simulink model "edrive"  (R2016b)
settings: Solver=ode1  StartTime=0.0  StopTime=1  FixedStep=ctrlConst.TsSim  MaxStep=1e-6  RelTol=1e-3  EnableMultiTasking=on
PreLoadFcn:
  | %rtwdemo_pmsmfoc_data
StartFcn:
  | %clear executionProfile
StopFcn:
  | %try
  | %  AddExecutionProfileToDataInspector();
  | %end
undefined symbols (not defined in the file or in its folder): canChannel, ctrlConst, ECM, EGM, hm11, hm13, hm5, hm7, Np, pmsm, sensors, sldrtexcb_modeswitch, SpdSetTest, theta0, TrqSetTest, Ts_10ms, Tsw
libraries: powerlib x26, canmsglib x23, simulink x14, canlib x12, powerlib_extras x9
(part 1 of 4)
Description:
  | Field-Oriented Control of Permanent Magnet Synchronous Machine
  | 
  | Demonstrates a Field-Oriented Control algorithm with Space Vector Modulation for a Permanent Magnet Synchronous Machine (PMSM).
  | The test bench can be used to evaluate the system performance. Examples include turning the motor on, searching for a valid rotor position,
  | transitioning to closed loop operation, and changing speed and torque during closed loop control.
  | The Embedded Processor subsystem contains the controller algorithm (which supports C code generation) as well as simulation models of peripherals.
settings Model: Creator=The MathWorks, Inc.  LastModifiedBy=xingchun.zhang
settings SolverCC: ZeroCrossControl=DisableAll  InsertRTBMode=Never (minimum delay)
settings DataIOCC: LimitDataPoints=on  SaveFormat=Array  SignalLogging=off  DSMLogging=off  ReturnWorkspaceOutputsName=effEDrive
settings OptimizationCC: DefaultParameterBehavior=Inlined  UseDivisionForNetSlopeComputation=on  UseFloatMulNetSlope=on  DefaultUnderspecifiedDataType=single  InlineInvariantSignals=on  PassReuseOutputArgsAs=Individual arguments  ExpressionDepthLimit=2147483647  ZeroExternalMemoryAtStartup=off  ZeroInternalMemoryAtStartup=off  NoFixptDivByZeroProtection=on  EfficientFloat2IntCast=on  LifeSpan=1
settings DebuggingCC: ReadBeforeWriteMsg=DisableAll  WriteAfterWriteMsg=DisableAll  WriteAfterReadMsg=DisableAll  AlgebraicLoopMsg=none  MultiTaskDSMMsg=warning  SingleTaskRateTransMsg=error  IntegerOverflowMsg=none  ParameterPrecisionLossMsg=none  FcnCallInpInsideContextMsg=warning  UnconnectedInputMsg=none  UnconnectedOutputMsg=none  UnconnectedLineMsg=none  BusObjectLabelMismatch=none  AssertControl=DisableAll  AllowSymbolicDim=off  StateNameClashWarn=warning  SFUnexpectedBacktrackingDiag=warning  SFNoUnconditionalDefaultTransitionDiag=warning  SFExecutionAtInitializationDiag=none  IntegerSaturationMsg=none  UnitsInconsistencyMsg=none
settings HardwareCC: ProdBitPerPointer=32  ProdBitPerSizeT=32  ProdBitPerPtrDiffT=32  ProdLargestAtomicFloat=None  ProdWordSize=32  ProdHWDeviceType=Infineon->TriCore
settings ModelReferenceCC: UpdateModelReferenceTargets=IfOutOfDate  ModelReferenceNumInstancesAllowed=Single  PropagateSignalLabelsOutOfModel=off
settings SFSimCC: SFSimEcho=off
settings RTWCC: SystemTargetFile=ert.tlc  GenerateMakefile=off  TemplateMakefile=ec_target.tmf  Description=Embedded Coder  GenerateReport=on  RTWVerbose=off  CustomInclude=C:\MatlabWS\motorcontrol\sfun  IncludeHyperlinkInReport=on  LaunchReport=on  PortableWordSizes=on  CodeExecutionProfiling=on  CodeProfilingSaveOptions=AllData  CodeProfilingInstrumentation=on  GenerateTraceInfo=on  GenerateTraceReport=on  GenerateTraceReportSl=on  GenerateTraceReportSf=on  GenerateTraceReportEml=on  GenerateWebview=on  GenerateCodeMetricsReport=on
settings RTWCC: CustomSource=|
  | C:\MatlabWS\motorcontrol\sfun\C2SfunShell.h
  | C:\MatlabWS\motorcontrol\sfun\C2SfunShell.c
settings CodeAppCC: ForceParamTrailComments=on  IgnoreCustomStorageClasses=off  IgnoreTestpoints=on  MaxIdLength=64  SimulinkDataObjDesc=on  MATLABFcnDesc=on  CustomSymbolStrGlobalVar=rt$N$M  CustomSymbolStrType=$N$M  CustomSymbolStrFcn=$N$M$F  CustomSymbolStrFcnArg=$I$N$M  CustomSymbolStrMacro=$N$M  InsertBlockDesc=on  MATLABSourceComments=on  InternalIdentifier=Classic
settings ERTTargetCC: GeneratePreprocessorConditionals=Disable all  CombineSignalStateStructs=on  SupportAbsoluteTime=off  SupportNonFinite=off  SupportComplex=off  SupportNonInlinedSFcns=on  RemoveResetFunc=off  ParenthesesLevel=Maximum  InlinedParameterPlacement=NonHierarchical  ERTCustomFileTemplate=example_file_process.tlc  ERTFilePackagingFormat=CompactWithDataFile  ConvertIfToSwitch=off  SuppressUnreachableDefaultCases=off
settings ConfigComp: CovMetricSettings=dcmtrzow  CovHTMLOptions=-aTS=1 -bRG=1 -bTC=1 -hTR=0 -nFC=0 -scm=1 -bcm=1 -xEv=0  CovHtmlReporting=on  CovSaveCumulativeToWorkspaceVar=on  CovSaveSingleToWorkspaceVar=on  CovExternalEMLEnable=off  CovSFcnEnable=off

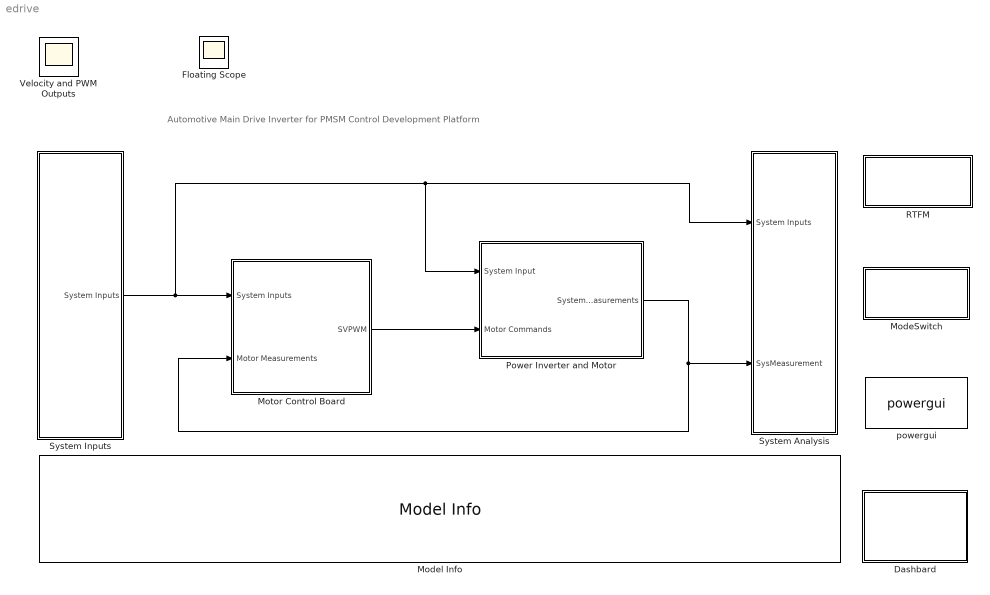
== system edrive ==
  note: Automotive Main Drive Inverter for PMSM Control
      | Development Platform
  Dashbard : Subsystem
  ModeSwitch : Subsystem  InitFcn=sldrtexcb_modeswitch('CheckKernel');  mask(Simulink Desktop Real-Time Example Mode Switch){}
      settings: OpenFcn=sldrtexcb_modeswitch(gcbh);
      mask Display: disp('Switch To\nExternal Mode');
  Model Info : simulink/Model-Wide Utilities/Model Info  Frame=on  DisplayStringWithTags=Model Description: %<Description>  HorizontalTextAlignment=Left  LeftAlignmentValue=0.02  SourceBlockDiagram=edrive  TagMaxNumber=20
  Motor Control Board : Subsystem
      mask Display: image('rtwdemo_pmsmfoc_processor.png')
  Power Inverter and Motor : Subsystem  Description=""
      mask Display: image('rtwdemo_pmsmfoc_motor.png')
  "RTFM " : Subsystem  mask(Simulink Desktop Real-Time Example Info){}
      settings: OpenFcn=web([docroot '/sldrt/examples/real-time-van-der-pol-simulation.html']);
      mask Display: disp('Info')
  System Analysis : Subsystem  Description=|
      | System Analysis for Speed Control Design
      | 
      | Analyize and plot signals used to analyize performance of
      | speed  control designs
      mask Display: fprintf('System\nAnalysis')
  System Inputs : Subsystem  Description=""  SystemSampleTime=10e-3
      mask Display: fprintf('System\nInputs')
  powergui : powerlib/powergui  Priority=1  SimulationMode=Discrete  SolverType=Tustin  SampleTime=ctrlConst.TsSimP  frequency=60  SPID=off  DisableSnubberDevices=off  DisableRonSwitches=off  DisableVfSwitches=off  SwTol=0  DisplayEquations=off  Interpol=off  ExternalGateDelay=off  methode=off  Ts=0  FunctionMessages=off  echomessages=off  HookPort=off  EnableUseOfTLC=off  x0status=blocks  frequencyindice=0  Pbase=100e6  ErrMax=1e-4  Iterations=50  UnitsV=kV  UnitsW=MW  buscounter=0  RestoreLinks=warning  ResistiveCurrentMeasurement=off  Frange=[0:2:500]  Ylog=off  Xlog=on  ShowGrid=off  save=off  variable=ZData  structure=ElecData  ZoomFFT=off  StartTime=0.482  cycles=10  DisplayStyle=2  fundamental=600  FreqAxis=off  MaxFrequency=10000  frequencyindicesteady=1  RmsSteady=1  display=off
  Floating Scope : Scope
  Velocity and PWM Outputs : Scope
  wires:
  Motor Control Board/1(SVPWM) -> Power Inverter and Motor/2(Motor Commands)
  System Inputs/1(System Inputs) -> Motor Control Board/1(System Inputs), System Analysis/1(System Inputs), Power Inverter and Motor/1(System Input)
  Power Inverter and Motor/1(System Measurements) -> Motor Control Board/2(Motor Measurements), System Analysis/2(SysMeasurement)

== system edrive/Dashbard ==
  Dashboard Scope : Subsystem  DialogController=hmiCreateDDGDialog  IsWebBlock=on  mask(MWDashboardBlock){webBlockId=dbaa0f85-305e-462e-a7a1-755dd39fbe0d, webBlockType=sdiscope, ShowInitialText=on, HMISrcModelName=edrive}
      mask prompts: webBlockId "WebBlock Id"; webBlockType "WebBlock Type"; HMISrcModelName "Source Model"
      mask help: SimulinkHMI:dialogs:HMIScopeDialogDesc
      mask Help: helpview([docroot '/mapfiles/simulink.map'], 'hmi_scope')
      mask Display:
      | if strcmp(get_param(bdroot(gcb),'BlockDiagramType'), 'library')
      |     image([(matlabroot) '/toolbox/simulink/hmi/icons/DashboardScope.png']);
      | end
  Gauge : Subsystem  DialogController=hmiCreateDDGDialog  IsWebBlock=on  mask(MWDashboardBlock){webBlockId=feaa2327-ad78-499e-96da-9991cfa67485, webBlockType=circulargauge, ShowInLibBrowser=on, ShowInitialText=on, HMISrcModelName=edrive}
      mask prompts: webBlockId "WebBlock Id"; webBlockType "WebBlock Type"; HMISrcModelName "Source Model"
      mask help: SimulinkHMI:dialogs:CircularGaugeDialogDesc
      mask Help: helpview([docroot '/mapfiles/simulink.map'], 'hmi_gauge')
      mask Display:
      | if strcmp(get_param(bdroot(gcb),'BlockDiagramType'), 'library')
      |     image([(matlabroot) '/toolbox/simulink/hmi/icons/CircularGauge.png']);
      | end
  Rotary Switch : Subsystem  DialogController=hmiCreateDDGDialog  IsWebBlock=on  mask(MWDashboardBlock){webBlockId=5f39aa38-4a9c-4792-be93-f8b3064abbd5, webBlockType=discreteknob, ShowInLibBrowser=on, ShowInitialText=on, HMISrcModelName=edrive}
      mask prompts: webBlockId "WebBlock Id"; webBlockType "WebBlock Type"; HMISrcModelName "Source Model"
      mask help: SimulinkHMI:dialogs:DiscreteKnobDialogDesc
      mask Help: helpview([docroot '/mapfiles/simulink.map'], 'hmi_rotary_switch')
      mask Display:
      | model = bdroot(gcb);
      | if strcmp(get_param(model,'BlockDiagramType'), 'library')
      |     image([(matlabroot) '/toolbox/simulink/hmi/icons/DiscreteKnob.png']);
      | end
  Slider : Subsystem  DialogController=hmiCreateDDGDialog  IsWebBlock=on  mask(MWDashboardBlock){webBlockId=79de6ff3-7337-4cfe-9aff-1e6db678eec5, webBlockType=slider, ShowInLibBrowser=on, ShowInitialText=on, HMISrcModelName=edrive}
      mask prompts: webBlockId "WebBlock Id"; webBlockType "WebBlock Type"; HMISrcModelName "Source Model"
      mask help: SimulinkHMI:dialogs:SliderDialogDesc
      mask Help: helpview([docroot '/mapfiles/simulink.map'], 'hmi_slider')
      mask Display:
      | if strcmp(get_param(bdroot(gcb),'BlockDiagramType'), 'library')
      |     image([(matlabroot) '/toolbox/simulink/hmi/icons/Slider.png']);
      | end

== system edrive/ModeSwitch ==

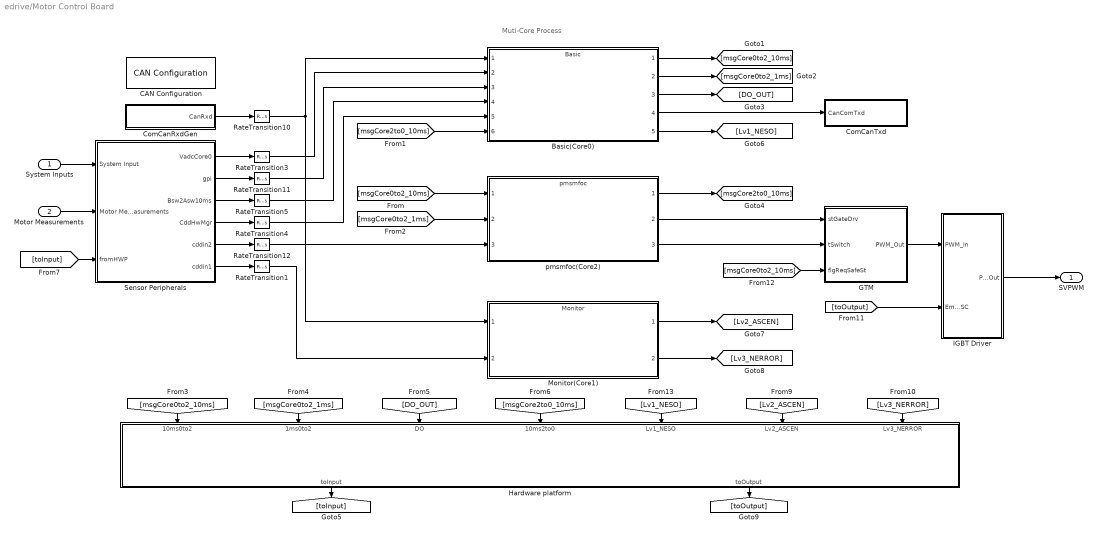
== system edrive/Motor Control Board ==
  note: Muti-Core Process
  System Inputs : Inport
  Motor Measurements : Inport  Port=2
  Basic(Core0) : ModelReference  ModelNameDialog=Basic.slx  SimulationMode=Normal  ModelReferenceVersion=1.11689
  CAN Configuration : canlib/CAN Configuration  BlockHandle=7528.001  DeviceMenu=(none)  Device=Kvaser Virtual 1 (Channel 1)  ObjConstructor=canChannel('Kvaser', 'Virtual 1', 1)  BusSpeed=500000  EnableBitParameters=off  SJW=1  TSEG1=4  TSEG2=3  NSamples=1  AckMode=Normal
  ComCanRxdGen : Subsystem
  ComCanTxd : Subsystem
  GTM : Subsystem  SystemSampleTime=Tsw
  Hardware platform : Subsystem  SystemSampleTime=Tsw
  IGBT Driver : Subsystem  SystemSampleTime=Tsw
  Monitor(Core1) : ModelReference  ModelNameDialog=Monitor.slx  SimulationMode=Normal  ModelReferenceVersion=1.8110
  RateTransition{1,3..5,10..12} (7 alike) : RateTransition
  Sensor Peripherals : Subsystem  Description=|
      | Elaborate Sensor Models
      | 
      | ADC and QEP and Encoder Models
  pmsmfoc(Core2) : ModelReference  ModelNameDialog=pmsmfoc.slx  SimulationMode=Normal  ModelReferenceVersion=1.9399
      settings: AttributesFormatString=|
      | -----------------------------
      | Sample rate: ctrlConst.TsSwitch
  SVPWM : Outport
  wires:
  System Inputs/1 -> Sensor Peripherals/1(System Input)
  Motor Measurements/1 -> Sensor Peripherals/2(Motor Measurements)
  ComCanRxdGen/1(CanRxd) -> RateTransition10/1
  Sensor Peripherals/2(gpi) -> RateTransition11/1
  Sensor Peripherals/5(cddin2) -> RateTransition12/1
  RateTransition12/1 -> pmsmfoc(Core2)/3
  RateTransition10/1 -> Monitor(Core1)/1, Basic(Core0)/1
  RateTransition11/1 -> Basic(Core0)/3
  pmsmfoc(Core2)/1 -> [msgCore2to0_10ms]
  pmsmfoc(Core2)/3 -> GTM/2(tSwitch)
  Basic(Core0)/1 -> [msgCore0to2_10ms]
  Sensor Peripherals/1(VadcCore0) -> RateTransition3/1
  Sensor Peripherals/6(cddin1) -> RateTransition1/1
  RateTransition1/1 -> Monitor(Core1)/2
  RateTransition3/1 -> Basic(Core0)/2
  [msgCore0to2_10ms] -> pmsmfoc(Core2)/1
  Basic(Core0)/2 -> [msgCore0to2_1ms]
  [msgCore0to2_1ms] -> pmsmfoc(Core2)/2
  [msgCore2to0_10ms] -> Basic(Core0)/6
  IGBT Driver/1(PWM_Out) -> SVPWM/1
  GTM/1(PWM_Out) -> IGBT Driver/1(PWM_In)
  Sensor Peripherals/4(CddHwMgr) -> RateTransition4/1
  RateTransition4/1 -> Basic(Core0)/5
  Sensor Peripherals/3(Bsw2Asw10ms) -> RateTransition5/1
  RateTransition5/1 -> Basic(Core0)/4
  pmsmfoc(Core2)/2 -> GTM/1(stGateDrv)
  Basic(Core0)/3 -> [DO_OUT]
  [msgCore0to2_10ms] -> Hardware platform/1(10ms0to2)
  [msgCore0to2_1ms] -> Hardware platform/2(1ms0to2)
  [DO_OUT] -> Hardware platform/3(DO)
  [msgCore2to0_10ms] -> Hardware platform/4(10ms2to0)
  Hardware platform/1(toInput) -> [toInput]
  [toInput] -> Sensor Peripherals/3(fromHWP)
  [Lv2_ASCEN] -> Hardware platform/6(Lv2_ASCEN)
  [Lv3_NERROR] -> Hardware platform/7(Lv3_NERROR)
  Hardware platform/2(toOutput) -> [toOutput]
  [toOutput] -> IGBT Driver/2(Emgy_ASC)
  [msgCore0to2_10ms] -> GTM/3(flgReqSafeSt)
  Basic(Core0)/4 -> ComCanTxd/1(CanComTxd)
  [Lv1_NESO] -> Hardware platform/5(Lv1_NESO)
  Basic(Core0)/5 -> [Lv1_NESO]
  Monitor(Core1)/1 -> [Lv2_ASCEN]
  Monitor(Core1)/2 -> [Lv3_NERROR]

== system edrive/Power Inverter and Motor ==
  note: Models the PMSM motor and inverter power electronics
      | Outputs electrical and mechanical measurements.
  note: Inverter and Motor
  System Input : Inport
  Motor Commands : Inport  Port=2
  Bus Creator : BusCreator  Inputs=3
  Bus Selector : BusSelector  OutputSignals=MotorMode,Load
  Inverter : Subsystem
  Motor_feishi150 : Subsystem
  System Measurements : Outport
  wires:
  Inverter/1("EleMeasurement ") -> Bus Creator/1  "electrical_measurements"
  Bus Creator/1 -> System Measurements/1
  Motor_feishi150/1(MotorMeasure) -> Bus Creator/2  "mechanical_measurements"
  System Input/1 -> Bus Selector/1
  Bus Selector/2 -> Motor_feishi150/2(Speed or Torque)  "<Load>"
  Motor Commands/1 -> Bus Creator/3, Inverter/1(gate1)
  Bus Selector/1 -> Motor_feishi150/1(MotorMode)  "<MotorMode>"
  connections:
  Motor_feishi150/LConn2 -- Inverter/RConn2
  Motor_feishi150/LConn1 -- Inverter/RConn1
  Motor_feishi150/LConn3 -- Inverter/RConn3

== system edrive/RTFM  ==

== system edrive/System Analysis ==
  note: System Analysis
  note: Visualize common signals of interest.
  System Inputs : Inport
  SysMeasurement : Inport  Port=2
  Bus Creator1 : BusCreator  Inputs=2
  Bus Selector4 : BusSelector  OutputSignals=Torque
  Data Type Conversion : DataTypeConversion  OutDataTypeStr=double
  Measure : Subsystem
  PMSM Drive : Scope  NumInputPorts=6
  Pass or not : Display
  System test : Subsystem
  effEDrive : Scope
  wires:
  SysMeasurement/1 -> Measure/1(motor)
  Bus Creator1/1 -> PMSM Drive/1, System test/1(torque_in)  "Torque"
  Measure/2(speed) -> PMSM Drive/2  "Speed"
  Measure/3(Current) -> PMSM Drive/3  "Is,iq,id"
  Measure/4(Voltage) -> PMSM Drive/4  "vs,vq,vd"
  Measure/5(Power) -> PMSM Drive/5  "Power"
  System test/1(Out) -> Pass or not/1
  System Inputs/1 -> Bus Selector4/1
  Bus Selector4/1 -> Data Type Conversion/1  "<Torque>"
  Measure/1(Torque) -> Bus Creator1/2  "TorqueAct"
  [ModeInCan] -> PMSM Drive/6
  Measure/6(effEDrive) -> effEDrive/1
  Data Type Conversion/1 -> Bus Creator1/1

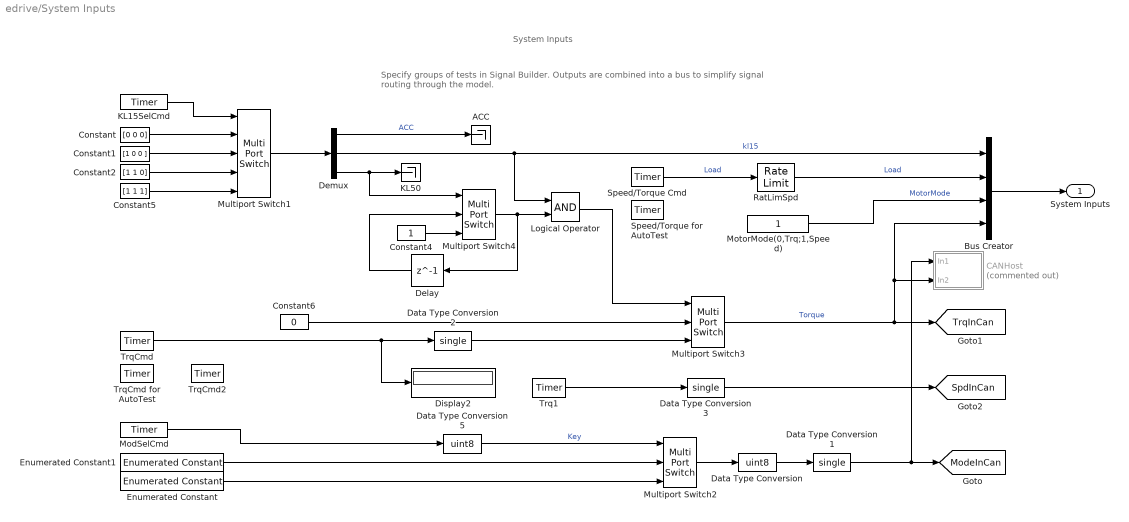
== system edrive/System Inputs ==
  note: System Inputs
  note: Specify groups of tests in Signal Builder. Outputs are combined into a bus
      | to simplify signal routing through the model.
  ACC : Terminator
  Bus Creator : BusCreator  Inputs=4
  CANHost : Subsystem  Commented=on
  Constant : Constant  Value=[0 0 0]  OutDataTypeStr=boolean
  Constant1 : Constant  Value=[1 0 0 ]  OutDataTypeStr=boolean
  Constant2 : Constant  Value=[1 1 0]  OutDataTypeStr=boolean
  Constant4 : Constant  OutDataTypeStr=boolean
  Constant5 : Constant  Value=[1 1 1]  OutDataTypeStr=boolean
  Constant6 : Constant  Value=0  OutDataTypeStr=single
  Data Type Conversion : DataTypeConversion  OutDataTypeStr=uint8
  Data Type Conversion1 : DataTypeConversion  OutDataTypeStr=single
  Data Type Conversion2 : DataTypeConversion  OutDataTypeStr=single
  Data Type Conversion3 : DataTypeConversion  OutDataTypeStr=single
  Data Type Conversion5 : DataTypeConversion  OutDataTypeStr=uint8  ConvertRealWorld=Stored Integer (SI)
  Delay : Delay  DelayLength=1  InitialCondition=0
  Demux : Demux  Outputs=3
  Display2 : Display
  Enumerated Constant : simulink/Sources/Enumerated Constant  OutDataTypeStr=Enum: ECM  Value=ECM.TrqCtrl  SampleTime=inf
  Enumerated Constant1 : simulink/Sources/Enumerated Constant  OutDataTypeStr=Enum: ECM  Value=ECM.Standby  SampleTime=inf
  KL15SelCmd : powerlib_extras/Control  Blocks/Timer  t="[ 0  0.03  0.1  0.2 0.9]"  e="[3  3  3  3 3]"
  KL50 : Terminator
  Logical Operator : Logic  AllPortsSameDT=off  OutDataTypeStr=boolean
  ModSelCmd : powerlib_extras/Control  Blocks/Timer  t="[ 0  0.1  0.2  0.3 0.4]"  e="[0  0  1  1 1]"
  MotorMode(0,Trq;1,Speed) : Constant  OutDataTypeStr=double
  Multiport Switch1 : MultiPortSwitch  DataPortOrder=Zero-based contiguous  Inputs=4
  Multiport Switch2 : MultiPortSwitch  DataPortOrder=Zero-based contiguous  Inputs=2
  Multiport Switch3 : MultiPortSwitch  DataPortOrder=Zero-based contiguous  Inputs=2
  Multiport Switch4 : MultiPortSwitch  DataPortOrder=Zero-based contiguous  Inputs=2
  RatLimSpd : RateLimiter  RisingSlewLimit=5000  FallingSlewLimit=-5000  LinearizeAsGain=off
  Speed/Torque Cmd : powerlib_extras/Control  Blocks/Timer  t="[ 0  0.05  0.25  0.4]"  e="[3  3  3  15]*(1000)"
  Speed/Torque for AutoTest : powerlib_extras/Control  Blocks/Timer  t="[ 0  0.1  0.25  0.5]"  e="[1  1  1  1]*SpdSetTest"
  Trq1 : powerlib_extras/Control  Blocks/Timer  t="[ 0  0.1  0.2  0.5]"  e="[0  0  2000  2000]*2"
  TrqCmd : powerlib_extras/Control  Blocks/Timer  t="[ 0  0.2 0.25 0.3 0.7 0.8]"  e="[ 0  0  0   1   1  1]*(200)"
  TrqCmd for AutoTest : powerlib_extras/Control  Blocks/Timer  t="[ 0  0.06  0.099 0.15]"  e="[ 0  1 1 1]*TrqSetTest"
  TrqCmd2 : powerlib_extras/Control  Blocks/Timer  t="[ 0  1  1.1  1.2 1.3 1.4 1.5 1.6 1.7 1.8 1.9 2.0 2.1 2.2 2.3 2.4 2.5 2.6 2.7 2.8 2.9]"  e=[ 0 1 2 3 4 5 6 7 8 9 10 11 12 13 14 15 16 17 18 19 20]*20
  System Inputs : Outport
  tag scope: ModeInCan=global, SpdInCan=global, TrqInCan=global
  wires:
  Constant/1 -> Multiport Switch1/2
  Multiport Switch1/1 -> Demux/1
  Enumerated Constant1/1 -> Multiport Switch2/2
  Multiport Switch2/1 -> Data Type Conversion/1
  Multiport Switch3/1 -> Bus Creator/4, CANHost/2(In2), [TrqInCan]  "Torque"
  Multiport Switch4/1 -> Logical Operator/2, Delay/1
  Delay/1 -> Multiport Switch4/2
  Constant4/1 -> Multiport Switch4/3
  Logical Operator/1 -> Multiport Switch3/1
  Constant1/1 -> Multiport Switch1/3
  Constant2/1 -> Multiport Switch1/4
  Demux/3 -> Multiport Switch4/1, KL50/1
  Demux/1 -> ACC/1  "ACC"
  Constant6/1 -> Multiport Switch3/2
  Demux/2 -> Bus Creator/1, Logical Operator/1  "kl15"
  Bus Creator/1 -> System Inputs/1
  Speed/Torque Cmd/1 -> RatLimSpd/1  "Load"
  Data Type Conversion/1 -> Data Type Conversion1/1
  Data Type Conversion1/1 -> CANHost/1(In1), [ModeInCan]
  Constant5/1 -> Multiport Switch1/5
  Data Type Conversion2/1 -> Multiport Switch3/3
  Trq1/1 -> Data Type Conversion3/1
  Data Type Conversion3/1 -> [SpdInCan]
  MotorMode(0,Trq;1,Speed)/1 -> Bus Creator/3  "MotorMode"
  RatLimSpd/1 -> Bus Creator/2  "Load"
  ModSelCmd/1 -> Data Type Conversion5/1
  Enumerated Constant/1 -> Multiport Switch2/3
  KL15SelCmd/1 -> Multiport Switch1/1
  Data Type Conversion5/1 -> Multiport Switch2/1  "Key"
  TrqCmd/1 -> Display2/1, Data Type Conversion2/1

== system edrive/Dashbard/Dashboard Scope ==

== system edrive/Dashbard/Gauge ==

== system edrive/Dashbard/Rotary Switch ==

== system edrive/Dashbard/Slider ==

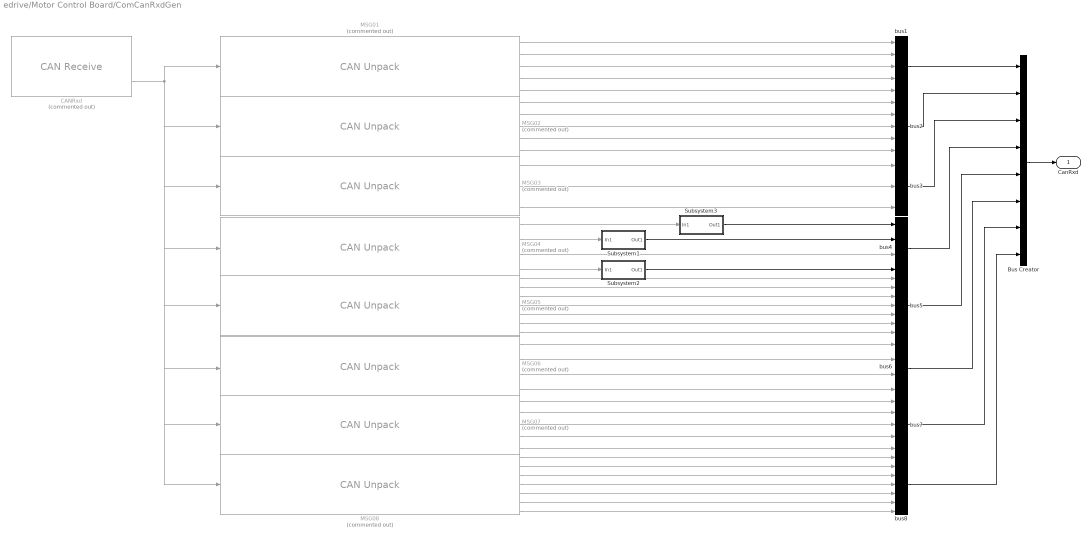
== system edrive/Motor Control Board/ComCanRxdGen ==
  Bus Creator : BusCreator  Inputs=8  OutDataTypeStr=Bus: CANRXDST
  CANRxd : canlib/CAN Receive  Commented=on  BlockHandle=7531.0005  DeviceMenu=Kvaser Virtual 1 (Channel 1)  Device=Kvaser Virtual 1 (Channel 1)  ObjConstructor=canChannel('Kvaser', 'Virtual 1', 1)  EnableStandardIDsFilter=off  StandardIDs=0  EnableExtendedIDsFilter=off  ExtendedIDs=0  SampleTime=0.01  MsgsPerTimestep=all  StdIDsCombo=Allow all  ExtIDsCombo=Allow all  InternalFilterUpdateStatus=off
  MSG01 : canmsglib/CAN Unpack  Commented=on  CANdbFile=C:\MatlabWS\motorcontrol\controller\CAN_COM.dbc  MsgList=MSG_01  MsgName=MSG_01  MsgIDType=Standard (11-bit identifier)  MsgIdentifier=768  MsgLength=8  SignalInfo=MSG01_IdcMax$0$0$0$4$4$4$4$4$4$4$#MSG01_IdcMin$0$0$0$4$4$4$4$4$4$4$#MSG01_UdcMax$0$0$0$4$4$4$4$4$4$4$#MSG01_UdcMin$0$0$0$4$4$4$4$4$4$4$#MSG01_stHvbMaiRly$0$0$0$4$4$4$4$4$4$4$#  NSignals=5  IDPort=off  TimestampPort=off  ErrorPort=off  RemotePort=off  LengthPort=off  StatusPort=off  StartBits=0  SignalSizes=0  ByteOrders=0  DataTypes=0  MultiplexTypes=0  MultiplexValues=0  Factors=0  Offsets=0  Minimums=0  Maximums=0
      settings: DataFormat=CANdb specified signals
  MSG02 : canmsglib/CAN Unpack  Commented=on  CANdbFile=C:\MatlabWS\motorcontrol\controller\CAN_COM.dbc  MsgList=MSG_02  MsgName=MSG_02  MsgIDType=Standard (11-bit identifier)  MsgIdentifier=784  MsgLength=8  SignalInfo=MSG02_KpHigh$0$0$0$4$4$4$4$4$4$4$#MSG02_KpLow$0$0$0$4$4$4$4$4$4$4$#MSG02_NDeltaBound$0$0$0$4$4$4$4$4$4$4$#MSG02_TrqPAmax$0$0$0$4$4$4$4$4$4$4$#MSG02_TrqPAmin$0$0$0$4$4$4$4$4$4$4$#  NSignals=5  IDPort=off  TimestampPort=off  ErrorPort=off  RemotePort=off  LengthPort=off  StatusPort=off  StartBits=0  SignalSizes=0  ByteOrders=0  DataTypes=0  MultiplexTypes=0  MultiplexValues=0  Factors=0  Offsets=0  Minimums=0  Maximums=0
      settings: DataFormat=CANdb specified signals
  MSG03 : canmsglib/CAN Unpack  Commented=on  CANdbFile=C:\MatlabWS\motorcontrol\controller\CAN_COM.dbc  MsgList=MSG_03  MsgName=MSG_03  MsgIDType=Standard (11-bit identifier)  MsgIdentifier=800  MsgLength=8  SignalInfo=MSG03_TrqMax$0$0$0$4$4$4$4$4$4$4$#MSG03_TrqMin$0$0$0$4$4$4$4$4$4$4$#MSG03_cTrqSlopeMax$0$0$0$4$4$4$4$4$4$4$#  NSignals=3  IDPort=off  TimestampPort=off  ErrorPort=off  RemotePort=off  LengthPort=off  StatusPort=off  StartBits=0  SignalSizes=0  ByteOrders=0  DataTypes=0  MultiplexTypes=0  MultiplexValues=0  Factors=0  Offsets=0  Minimums=0  Maximums=0
      settings: DataFormat=CANdb specified signals
  MSG04 : canmsglib/CAN Unpack  Commented=on  CANdbFile=C:\MatlabWS\motorcontrol\controller\CAN_COM.dbc  MsgList=MSG_04  MsgName=MSG_04  MsgIDType=Standard (11-bit identifier)  MsgIdentifier=256  MsgLength=8  SignalInfo=MSG04_NSetP$0$0$0$4$4$4$4$4$4$4$#MSG04_TrqSetP$0$0$0$4$4$4$4$4$4$4$#MSG04_UdcSetP$0$0$0$4$4$4$4$4$4$4$#MSG04_stModeReq$0$0$0$4$4$4$4$4$4$4$#  NSignals=4  IDPort=off  TimestampPort=off  ErrorPort=off  RemotePort=off  LengthPort=off  StatusPort=off  StartBits=0  SignalSizes=0  ByteOrders=0  DataTypes=0  MultiplexTypes=0  MultiplexValues=0  Factors=0  Offsets=0  Minimums=0  Maximums=0
      settings: DataFormat=CANdb specified signals
  MSG05 : canmsglib/CAN Unpack  Commented=on  CANdbFile=C:\MatlabWS\motorcontrol\controller\CAN_COM.dbc  MsgList=MSG_05  MsgName=MSG_05  MsgIDType=Standard (11-bit identifier)  MsgIdentifier=272  MsgLength=8  SignalInfo=MSG05_FrqStrSetP$0$0$0$4$4$4$4$4$4$4$#MSG05_IsSetP$0$0$0$4$4$4$4$4$4$4$#MSG05_OfsAl$0$0$0$4$4$4$4$4$4$4$#MSG05_PumpCtl$0$0$0$4$4$4$4$4$4$4$#MSG05_bSetOfsAl$0$0$0$4$4$4$4$4$4$4$#MSG05_bUseFrqStrSynt$0$0$0$4$4$4$4$4$4$4$#MSG05_flgInvrCanActvnCmd$0$0$0$4$4$4$4$4$4$4$#  NSignals=7  IDPort=off  TimestampPort=off  ErrorPort=off  RemotePort=off  LengthPort=off  StatusPort=off  StartBits=0  SignalSizes=0  ByteOrders=0  DataTypes=0  MultiplexTypes=0  MultiplexValues=0  Factors=0  Offsets=0  Minimums=0  Maximums=0
      settings: DataFormat=CANdb specified signals
  MSG06 : canmsglib/CAN Unpack  Commented=on  CANdbFile=C:\MatlabWS\motorcontrol\controller\CAN_COM.dbc  MsgList=MSG_06  MsgName=MSG_06  MsgIDType=Standard (11-bit identifier)  MsgIdentifier=288  MsgLength=8  SignalInfo=MSG06_TrqDmpLim$0$0$0$4$4$4$4$4$4$4$#MSG06_TrqDmpMax$0$0$0$4$4$4$4$4$4$4$#MSG06_kDmp$0$0$0$4$4$4$4$4$4$4$#MSG06_stDstCReq$0$0$0$4$4$4$4$4$4$4$#  NSignals=4  IDPort=off  TimestampPort=off  ErrorPort=off  RemotePort=off  LengthPort=off  StatusPort=off  StartBits=0  SignalSizes=0  ByteOrders=0  DataTypes=0  MultiplexTypes=0  MultiplexValues=0  Factors=0  Offsets=0  Minimums=0  Maximums=0
      settings: DataFormat=CANdb specified signals
  MSG07 : canmsglib/CAN Unpack  Commented=on  CANdbFile=C:\MatlabWS\motorcontrol\controller\CAN_COM.dbc  MsgList=MSG_07  MsgName=CAN Msg  MsgIDType=Standard (11-bit identifier)  MsgIdentifier=0  MsgLength=8  SignalInfo=MSG07_IdcHvSetP$0$0$0$4$4$4$4$4$4$4$#MSG07_IdcLvSetP$0$0$0$4$4$4$4$4$4$4$#MSG07_UdcHvSetP$0$0$0$4$4$4$4$4$4$4$#MSG07_UdcLvSetP$0$0$0$4$4$4$4$4$4$4$#MSG07_stModeReq$0$0$0$4$4$4$4$4$4$4$#  NSignals=5  IDPort=off  TimestampPort=off  ErrorPort=off  RemotePort=off  LengthPort=off  StatusPort=off  StartBits=0  SignalSizes=0  ByteOrders=0  DataTypes=0  MultiplexTypes=0  MultiplexValues=0  Factors=0  Offsets=0  Minimums=0  Maximums=0
      settings: DataFormat=CANdb specified signals
  MSG08 : canmsglib/CAN Unpack  Commented=on  CANdbFile=C:\MatlabWS\motorcontrol\controller\CAN_COM.dbc  MsgList=MSG_08  MsgName=CAN Msg  MsgIDType=Standard (11-bit identifier)  MsgIdentifier=0  MsgLength=8  SignalInfo=MSG08_Alpha_Voltage_Cmd$0$0$0$4$4$4$4$4$4$4$#MSG08_Beta_Voltage_Cmd$0$0$0$4$4$4$4$4$4$4$#MSG08_D_Current_Cmd$0$0$0$4$4$4$4$4$4$4$#MSG08_D_Voltage_Cmd$0$0$0$4$4$4$4$4$4$4$#MSG08_Q_Current_Cmd$0$0$0$4$4$4$4$4$4$4$#MSG08_Q_Volatge_Cmd$0$0$0$4$4$4$4$4$4$4$#MSG08_control_mode$0$0$0$4$4$4$4$4$4$4$#  NSignals=7  IDPort=off  TimestampPort=off  ErrorPort=off  RemotePort=off  LengthPort=off  StatusPort=off  StartBits=0  SignalSizes=0  ByteOrders=0  DataTypes=0  MultiplexTypes=0  MultiplexValues=0  Factors=0  Offsets=0  Minimums=0  Maximums=0
      settings: DataFormat=CANdb specified signals
  Subsystem1 : Subsystem
  Subsystem2 : Subsystem
  Subsystem3 : Subsystem
  bus1 : BusCreator  Inputs=5  OutDataTypeStr=Bus: msg_MSG_01
  bus2 : BusCreator  Inputs=5  OutDataTypeStr=Bus: msg_MSG_02
  bus3 : BusCreator  Inputs=3  OutDataTypeStr=Bus: msg_MSG_03
  bus4 : BusCreator  Inputs=4  OutDataTypeStr=Bus: msg_MSG_04
  bus5 : BusCreator  Inputs=7  OutDataTypeStr=Bus: msg_MSG_05
  bus6 : BusCreator  Inputs=4  OutDataTypeStr=Bus: msg_MSG_06
  bus7 : BusCreator  Inputs=5  OutDataTypeStr=Bus: msg_MSG_07
  bus8 : BusCreator  Inputs=7  OutDataTypeStr=Bus: msg_MSG_08
  CanRxd : Outport  OutDataTypeStr=Bus: CANRXDST
  wires:
  Bus Creator/1 -> CanRxd/1
  MSG01/1 -> bus1/1
  MSG01/2 -> bus1/2
  MSG01/3 -> bus1/3
  MSG01/4 -> bus1/4
  MSG01/5 -> bus1/5
  CANRxd/2 -> MSG01/1, MSG02/1, MSG03/1, MSG04/1, MSG05/1, MSG06/1, MSG07/1, MSG08/1
  MSG02/1 -> bus2/1
  MSG02/2 -> bus2/2
  MSG02/3 -> bus2/3
  MSG02/4 -> bus2/4
  MSG02/5 -> bus2/5
  MSG03/1 -> bus3/1
  MSG03/2 -> bus3/2
  MSG04/1 -> Subsystem3/1(In1)
  MSG04/2 -> Subsystem1/1(In1)
  MSG04/3 -> bus4/3
  MSG04/4 -> Subsystem2/1(In1)
  MSG05/1 -> bus5/1
  MSG05/2 -> bus5/2
  MSG05/3 -> bus5/3
  MSG05/4 -> bus5/4
  MSG05/5 -> bus5/5
  MSG05/6 -> bus5/6
  MSG05/7 -> bus5/7
  MSG06/1 -> bus6/1
  MSG06/2 -> bus6/2
  MSG06/3 -> bus6/3
  MSG06/4 -> bus6/4
  MSG07/1 -> bus7/1
  MSG07/2 -> bus7/2
  MSG07/3 -> bus7/3
  MSG07/4 -> bus7/4
  MSG07/5 -> bus7/5
  MSG08/1 -> bus8/1
  MSG08/2 -> bus8/2
  MSG08/3 -> bus8/3
  MSG08/4 -> bus8/4
  MSG08/5 -> bus8/5
  MSG08/6 -> bus8/6
  MSG08/7 -> bus8/7
  MSG03/3 -> bus3/3
  Subsystem1/1(Out1) -> bus4/2
  Subsystem2/1(Out1) -> bus4/4
  bus1/1 -> Bus Creator/1
  bus2/1 -> Bus Creator/2
  bus3/1 -> Bus Creator/3
  bus4/1 -> Bus Creator/4
  bus5/1 -> Bus Creator/5
  bus6/1 -> Bus Creator/6
  bus7/1 -> Bus Creator/7
  bus8/1 -> Bus Creator/8
  Subsystem3/1(Out1) -> bus4/1

== system edrive/Motor Control Board/ComCanTxd ==
  CanComTxd : Inport  OutDataTypeStr=Bus: CANTXDST  SampleTime=Ts_10ms
  Bus Selector1 : BusSelector  OutputSignals=msg_EM_01,msg_EM_02,msg_EM_03,msg_EM_04,msg_EM_05,msg_EM_06,msg_EM_07
  Bus Selector2 : BusSelector  OutputSignals=EM01_IdcCurr,EM01_IsCurr,EM01_NCurr,EM01_TrqCurr,EM01_UdcCurr,EM01_stMode
  Bus Selector3 : BusSelector  OutputSignals=EM02_DBCTempU,EM02_DBCTempV,EM02_DBCTempW,EM02_TempCurrIGBT,EM02_TempCurrMot,EM02_TempCurrRotor,EM02_UT30Curr,EM02_bDernOvrIdc,EM02_bDernOvrUdc,EM02_bDernTemp,EM02_bDernTrqMax,EM02_bDernTrqMin,EM02_bDernUndrIdc,EM02_bDernUndrUdc,EM02_bDiagReq,EM02_bDstCActv,EM02_bReadyHv
  Bus Selector4 : BusSelector  OutputSignals=EM03_TempCurrCool,EM03_TempCurrDde,EM03_TrqAbsMax,EM03_TrqAbsMin,EM03_TrqCurrWoDstC,EM03_stGateDrv,EM03_stTrqEmMax,EM03_stTrqEmMin
  Bus Selector5 : BusSelector  OutputSignals=EM04_Isd,EM04_Isq,EM04_OfsAl,EM04_TempCurrPCB,EM04_agRtrElecSnsr
  Bus Selector6 : BusSelector  OutputSignals=EM05_FailCode1,EM05_FailCode2,EM05_FailCode3,EM05_FailCode4
  Bus Selector7 : BusSelector  OutputSignals=EM06_CodeVer,EM06_DataVer
  Bus Selector8 : BusSelector  OutputSignals=EM07_InterlockVtg,EM07_NCANSet,EM07_PumpVtg
  CAN Transmit : canlib/CAN Transmit  BlockHandle=7641.0006  DeviceMenu=(none)  Device=Kvaser Virtual 1 (Channel 1)  ObjConstructor=canChannel('Kvaser', 'Virtual 1', 1)  EnablePeriodicTransmit=off  MessagePeriod=1.000
  EM1 : canmsglib/CAN Pack  CANdbFile=C:\MatlabWS\motorcontrol\controller\CAN_COM.dbc  MsgList=EM_01  MsgName=EM_01  MsgIDType=Standard (11-bit identifier)  MsgIdentifier=512  MsgLength=8  SignalInfo=EM01_IdcCurr$32$11$1$2$1$0$1$-1023$-1023$1024$#EM01_IsCurr$53$11$1$2$1$0$5.000000e-01$0$0$1.023500e+03$#EM01_NCurr$16$16$1$2$1$0$1$-32767$-32767$32768$#EM01_TrqCurr$0$11$1$2$1$0$1$-1023$-1023$1024$#EM01_UdcCurr$43$10$1$2$1$0$1$0$0$1023$#EM01_stMode$11$4$1$2$1$0$1$0$0$15$#  NSignals=6  StartBits=str2num('[int32(32);int32(53);int32(16);int32(0);int32(43);int32(11)]')  SignalSizes=str2num('[int32(11);int32(11);int32(16);int32(11);int32(10);int32(4)]')  ByteOrders=str2num('[int32(1);int32(1);int32(1);int32(1);int32(1);int32(1)]')  DataTypes=str2num('[int32(2);int32(2);int32(2);int32(2);int32(2);int32(2)]')  MultiplexTypes=str2num('[int32(1);int32(1);int32(1);int32(1);int32(1);int32(1)]')  MultiplexValues=str2num('[double(0);double(0);double(0);double(0);double(0);double(0)]')  Factors=str2num('[double(1);double(5.000000e-01);double(1);double(1);double(1);double(1)]')  Offsets=str2num('[double(-1023);double(0);double(-32767);double(-1023);double(0);double(0)]')  Minimums=str2num('[double(-1023);double(0);double(-32767);double(-1023);double(0);double(0)]')  Maximums=str2num('[double(1024);double(1.023500e+03);double(32768);double(1024);double(1023);double(15)]')  Remote=off
      settings: DataFormat=CANdb specified signals
  EM2 : canmsglib/CAN Pack  CANdbFile=C:\MatlabWS\motorcontrol\controller\CAN_COM.dbc  MsgList=EM_02  MsgName=EM_02  MsgIDType=Standard (11-bit identifier)  MsgIdentifier=1024  MsgLength=8  SignalInfo=EM02_DBCTempU$24$8$1$2$1$0$1$-40$-40$215$#EM02_DBCTempV$32$8$1$2$1$0$1$-40$-40$215$#EM02_DBCTempW$40$8$1$2$1$0$1$-40$-40$215$#EM02_TempCurrIGBT$16$8$1$2$1$0$1$-40$-40$215$#EM02_TempCurrMot$0$8$1$2$1$0$1$-40$-40$215$#EM02_TempCurrRotor$8$8$1$2$1$0$1$-40$-40$215$#EM02_UT30Curr$58$6$1$2$1$0$5.000000e-01$0$0$3.150000e+01$#EM02_bDernOvrIdc$50$1$1$2$1$0$1$0$0$1$#EM02_bDernOvrUdc$48$1$1$2$1$0$1$0$0$1$#EM02_bDernTemp$52$1$1$2$1$0$1$0$0$1$#EM02_bDernTrqMax$55$1$1$2$1$0$1$0$0$1$#EM02_bDernTrqMin$54$1$1$2$1$0$1$0$0$1$#EM02_bDernUndrIdc$51$1$1$2$1$0$1$0$0$1$#EM02_bDernUndrUdc$49$1$1$2$1$0$1$0$0$1$#EM02_bDiagReq$53$1$1$2$1$0$1$0$0$1$#EM02_bDstCActv$56$1$1$2$1$0$1$0$0$1$#EM02_bReadyHv$57$1$1$2$1$0$1$0$0$1$#  NSignals=17  StartBits=str2num('[int32(24);int32(32);int32(40);int32(16);int32(0);int32(8);int32(58);int32(50);int32(48);int32(52);int32(55);int32(54);int32(51);int32(49);int32(53);int32(56);int32(57)]')  SignalSizes=str2num('[int32(8);int32(8);int32(8);int32(8);int32(8);int32(8);int32(6);int32(1);int32(1);int32(1);int32(1);int32(1);int32(1);int32(1);int32(1);int32(1);int32(1)]')  ByteOrders=str2num('[int32(1);int32(1);int32(1);int32(1);int32(1);int32(1);int32(1);int32(1);int32(1);int32(1);int32(1);int32(1);int32(1);int32(1);int32(1);int32(1);int32(1)]')  DataTypes=str2num('[int32(2);int32(2);int32(2);int32(2);int32(2);int32(2);int32(2);int32(2);int32(2);int32(2);int32(2);int32(2);int32(2);int32(2);int32(2);int32(2);int32(2)]')  MultiplexTypes=str2num('[int32(1);int32(1);int32(1);int32(1);int32(1);int32(1);int32(1);int32(1);int32(1);int32(1);int32(1);int32(1);int32(1);int32(1);int32(1);int32(1);int32(1)]')  MultiplexValues=str2num('[double(0);double(0);double(0);double(0);double(0);double(0);double(0);double(0);double(0);double(0);double(0);double(0);double(0);double(0);double(0);double(0);double(0)]')  Factors=str2num('[double(1);double(1);double(1);double(1);double(1);double(1);double(5.000000e-01);double(1);double(1);double(1);double(1);double(1);double(1);double(1);double(1);double(1);double(1)]')  Offsets=str2num('[double(-40);double(-40);double(-40);double(-40);double(-40);double(-40);double(0);double(0);double(0);double(0);double(0);double(0);double(0);double(0);double(0);double(0);double(0)]')  Minimums=str2num('[double(-40);double(-40);double(-40);double(-40);double(-40);double(-40);double(0);double(0);double(0);double(0);double(0);double(0);double(0);double(0);double(0);double(0);double(0)]')  Maximums=str2num('[double(215);double(215);double(215);double(215);double(215);double(215);double(3.150000e+01);double(1);double(1);double(1);double(1);double(1);double(1);double(1);double(1);double(1);double(1)]')  Remote=off
      settings: DataFormat=CANdb specified signals
  EM3 : canmsglib/CAN Pack  CANdbFile=C:\MatlabWS\motorcontrol\controller\CAN_COM.dbc  MsgList=EM_03  MsgName=EM_03  MsgIDType=Standard (11-bit identifier)  MsgIdentifier=528  MsgLength=8  SignalInfo=EM03_TempCurrCool$48$8$1$2$1$0$1$-40$-40$215$#EM03_TempCurrDde$56$8$1$2$1$0$1$-40$-40$215$#EM03_TrqAbsMax$0$11$1$2$1$0$1$-1023$-1023$1024$#EM03_TrqAbsMin$11$11$1$2$1$0$1$-1023$-1023$1024$#EM03_TrqCurrWoDstC$24$11$1$2$1$0$1$-1023$-1023$1024$#EM03_stGateDrv$22$2$1$2$1$0$1$0$0$3$#EM03_stTrqEmMax$35$6$1$2$1$0$1$0$0$23$#EM03_stTrqEmMin$41$6$1$2$1$0$1$0$0$23$#  NSignals=8  StartBits=str2num('[int32(48);int32(56);int32(0);int32(11);int32(24);int32(22);int32(35);int32(41)]')  SignalSizes=str2num('[int32(8);int32(8);int32(11);int32(11);int32(11);int32(2);int32(6);int32(6)]')  ByteOrders=str2num('[int32(1);int32(1);int32(1);int32(1);int32(1);int32(1);int32(1);int32(1)]')  DataTypes=str2num('[int32(2);int32(2);int32(2);int32(2);int32(2);int32(2);int32(2);int32(2)]')  MultiplexTypes=str2num('[int32(1);int32(1);int32(1);int32(1);int32(1);int32(1);int32(1);int32(1)]')  MultiplexValues=str2num('[double(0);double(0);double(0);double(0);double(0);double(0);double(0);double(0)]')  Factors=str2num('[double(1);double(1);double(1);double(1);double(1);double(1);double(1);double(1)]')  Offsets=str2num('[double(-40);double(-40);double(-1023);double(-1023);double(-1023);double(0);double(0);double(0)]')  Minimums=str2num('[double(-40);double(-40);double(-1023);double(-1023);double(-1023);double(0);double(0);double(0)]')  Maximums=str2num('[double(215);double(215);double(1024);double(1024);double(1024);double(3);double(23);double(23)]')  Remote=off
      settings: DataFormat=CANdb specified signals
  EM4 : canmsglib/CAN Pack  CANdbFile=C:\MatlabWS\motorcontrol\controller\CAN_COM.dbc  MsgList=EM_04  MsgName=EM_04  MsgIDType=Standard (11-bit identifier)  MsgIdentifier=560  MsgLength=8  SignalInfo=EM04_Isd$12$12$1$2$1$0$5.000000e-01$-1.023500e+03$-1.023500e+03$1024$#EM04_Isq$24$12$1$2$1$0$5.000000e-01$-1.023500e+03$-1.023500e+03$1024$#EM04_OfsAl$0$12$1$2$1$0$8.789063e-02$0$0$3.599121e+02$#EM04_TempCurrPCB$40$8$1$2$1$0$1$-40$-40$215$#EM04_agRtrElecSnsr$48$12$1$2$1$0$8.789063e-02$0$0$3.599121e+02$#  NSignals=5  StartBits=str2num('[int32(12);int32(24);int32(0);int32(40);int32(48)]')  SignalSizes=str2num('[int32(12);int32(12);int32(12);int32(8);int32(12)]')  ByteOrders=str2num('[int32(1);int32(1);int32(1);int32(1);int32(1)]')  DataTypes=str2num('[int32(2);int32(2);int32(2);int32(2);int32(2)]')  MultiplexTypes=str2num('[int32(1);int32(1);int32(1);int32(1);int32(1)]')  MultiplexValues=str2num('[double(0);double(0);double(0);double(0);double(0)]')  Factors=str2num('[double(5.000000e-01);double(5.000000e-01);double(8.789063e-02);double(1);double(8.789063e-02)]')  Offsets=str2num('[double(-1.023500e+03);double(-1.023500e+03);double(0);double(-40);double(0)]')  Minimums=str2num('[double(-1.023500e+03);double(-1.023500e+03);double(0);double(-40);double(0)]')  Maximums=str2num('[double(1024);double(1024);double(3.599121e+02);double(215);double(3.599121e+02)]')  Remote=off
      settings: DataFormat=CANdb specified signals
  EM5 : canmsglib/CAN Pack  CANdbFile=C:\MatlabWS\motorcontrol\controller\CAN_COM.dbc  MsgList=EM_05  MsgName=EM_05  MsgIDType=Standard (11-bit identifier)  MsgIdentifier=576  MsgLength=8  SignalInfo=EM05_FailCode1$0$16$1$2$1$0$1$0$0$65535$#EM05_FailCode2$16$16$1$2$1$0$1$0$0$65535$#EM05_FailCode3$32$16$1$2$1$0$1$0$0$65535$#EM05_FailCode4$48$16$1$2$1$0$1$0$0$65535$#  NSignals=4  StartBits=str2num('[int32(0);int32(16);int32(32);int32(48)]')  SignalSizes=str2num('[int32(16);int32(16);int32(16);int32(16)]')  ByteOrders=str2num('[int32(1);int32(1);int32(1);int32(1)]')  DataTypes=str2num('[int32(2);int32(2);int32(2);int32(2)]')  MultiplexTypes=str2num('[int32(1);int32(1);int32(1);int32(1)]')  MultiplexValues=str2num('[double(0);double(0);double(0);double(0)]')  Factors=str2num('[double(1);double(1);double(1);double(1)]')  Offsets=str2num('[double(0);double(0);double(0);double(0)]')  Minimums=str2num('[double(0);double(0);double(0);double(0)]')  Maximums=str2num('[double(65535);double(65535);double(65535);double(65535)]')  Remote=off
      settings: DataFormat=CANdb specified signals
  EM6 : canmsglib/CAN Pack  CANdbFile=C:\MatlabWS\motorcontrol\controller\CAN_COM.dbc  MsgList=EM_06  MsgName=EM_06  MsgIDType=Standard (11-bit identifier)  MsgIdentifier=1056  MsgLength=8  SignalInfo=EM06_CodeVer$0$32$1$2$1$0$1$0$0$4294967295$#EM06_DataVer$32$32$1$2$1$0$1$0$0$4294967295$#  NSignals=2  StartBits=str2num('[int32(0);int32(32)]')  SignalSizes=str2num('[int32(32);int32(32)]')  ByteOrders=str2num('[int32(1);int32(1)]')  DataTypes=str2num('[int32(2);int32(2)]')  MultiplexTypes=str2num('[int32(1);int32(1)]')  MultiplexValues=str2num('[double(0);double(0)]')  Factors=str2num('[double(1);double(1)]')  Offsets=str2num('[double(0);double(0)]')  Minimums=str2num('[double(0);double(0)]')  Maximums=str2num('[double(4294967295);double(4294967295)]')  Remote=off
      settings: DataFormat=CANdb specified signals
  EM7 : canmsglib/CAN Pack  CANdbFile=C:\MatlabWS\motorcontrol\controller\CAN_COM.dbc  MsgList=EM_07  MsgName=EM_07  MsgIDType=Standard (11-bit identifier)  MsgIdentifier=624  MsgLength=8  SignalInfo=EM07_InterlockVtg$8$8$1$2$1$0$2.000000e-02$0$0$5$#EM07_NCANSet$16$16$1$2$1$0$1$-32767$-32767$32768$#EM07_PumpVtg$0$8$1$2$1$0$2.000000e-02$0$0$5$#  NSignals=3  StartBits=str2num('[int32(8);int32(16);int32(0)]')  SignalSizes=str2num('[int32(8);int32(16);int32(8)]')  ByteOrders=str2num('[int32(1);int32(1);int32(1)]')  DataTypes=str2num('[int32(2);int32(2);int32(2)]')  MultiplexTypes=str2num('[int32(1);int32(1);int32(1)]')  MultiplexValues=str2num('[double(0);double(0);double(0)]')  Factors=str2num('[double(2.000000e-02);double(1);double(2.000000e-02)]')  Offsets=str2num('[double(0);double(-32767);double(0)]')  Minimums=str2num('[double(0);double(-32767);double(0)]')  Maximums=str2num('[double(5);double(32768);double(5)]')  Remote=off
      settings: DataFormat=CANdb specified signals
  Mux : Mux  Inputs=7
  wires:
  EM1/1 -> Mux/1
  Mux/1 -> CAN Transmit/1
  EM2/1 -> Mux/2
  EM3/1 -> Mux/3
  EM7/1 -> Mux/7
  EM4/1 -> Mux/4
  EM6/1 -> Mux/6
  EM5/1 -> Mux/5
  CanComTxd/1 -> Bus Selector1/1
  Bus Selector1/1 -> Bus Selector2/1  "<msg_EM_01>"
  Bus Selector2/1 -> EM1/1  "<EM01_IdcCurr>"
  Bus Selector2/2 -> EM1/2  "<EM01_IsCurr>"
  Bus Selector2/3 -> EM1/3  "<EM01_NCurr>"
  Bus Selector2/4 -> EM1/4  "<EM01_TrqCurr>"
  Bus Selector2/5 -> EM1/5  "<EM01_UdcCurr>"
  Bus Selector2/6 -> EM1/6  "<EM01_stMode>"
  Bus Selector1/2 -> Bus Selector3/1  "<msg_EM_02>"
  Bus Selector3/14 -> EM2/14  "<EM02_bDernUndrUdc>"
  Bus Selector3/8 -> EM2/8  "<EM02_bDernOvrIdc>"
  Bus Selector3/17 -> EM2/17  "<EM02_bReadyHv>"
  Bus Selector3/13 -> EM2/13  "<EM02_bDernUndrIdc>"
  Bus Selector3/7 -> EM2/7  "<EM02_UT30Curr>"
  Bus Selector3/12 -> EM2/12  "<EM02_bDernTrqMin>"
  Bus Selector3/11 -> EM2/11  "<EM02_bDernTrqMax>"
  Bus Selector3/9 -> EM2/9  "<EM02_bDernOvrUdc>"
  Bus Selector3/10 -> EM2/10  "<EM02_bDernTemp>"
  Bus Selector3/15 -> EM2/15  "<EM02_bDiagReq>"
  Bus Selector3/16 -> EM2/16  "<EM02_bDstCActv>"
  Bus Selector3/5 -> EM2/5  "<EM02_TempCurrMot>"
  Bus Selector3/1 -> EM2/1  "<EM02_DBCTempU>"
  Bus Selector3/6 -> EM2/6  "<EM02_TempCurrRotor>"
  Bus Selector3/3 -> EM2/3  "<EM02_DBCTempW>"
  Bus Selector3/2 -> EM2/2  "<EM02_DBCTempV>"
  Bus Selector3/4 -> EM2/4  "<EM02_TempCurrIGBT>"
  Bus Selector1/3 -> Bus Selector4/1  "<msg_EM_03>"
  Bus Selector4/3 -> EM3/3  "<EM03_TrqAbsMax>"
  Bus Selector4/2 -> EM3/2  "<EM03_TempCurrDde>"
  Bus Selector4/5 -> EM3/5  "<EM03_TrqCurrWoDstC>"
  Bus Selector4/6 -> EM3/6  "<EM03_stGateDrv>"
  Bus Selector4/4 -> EM3/4  "<EM03_TrqAbsMin>"
  Bus Selector4/7 -> EM3/7  "<EM03_stTrqEmMax>"
  Bus Selector4/1 -> EM3/1  "<EM03_TempCurrCool>"
  Bus Selector4/8 -> EM3/8  "<EM03_stTrqEmMin>"
  Bus Selector1/4 -> Bus Selector5/1  "<msg_EM_04>"
  Bus Selector5/1 -> EM4/1  "<EM04_Isd>"
  Bus Selector5/3 -> EM4/3  "<EM04_OfsAl>"
  Bus Selector5/2 -> EM4/2  "<EM04_Isq>"
  Bus Selector5/5 -> EM4/5  "<EM04_agRtrElecSnsr>"
  Bus Selector5/4 -> EM4/4  "<EM04_TempCurrPCB>"
  Bus Selector1/5 -> Bus Selector6/1  "<msg_EM_05>"
  Bus Selector6/4 -> EM5/4  "<EM05_FailCode4>"
  Bus Selector6/2 -> EM5/2  "<EM05_FailCode2>"
  Bus Selector6/3 -> EM5/3  "<EM05_FailCode3>"
  Bus Selector6/1 -> EM5/1  "<EM05_FailCode1>"
  Bus Selector1/6 -> Bus Selector7/1  "<msg_EM_06>"
  Bus Selector7/1 -> EM6/1  "<EM06_CodeVer>"
  Bus Selector7/2 -> EM6/2  "<EM06_DataVer>"
  Bus Selector1/7 -> Bus Selector8/1  "<msg_EM_07>"
  Bus Selector8/3 -> EM7/3  "<EM07_PumpVtg>"
  Bus Selector8/2 -> EM7/2  "<EM07_NCANSet>"
  Bus Selector8/1 -> EM7/1  "<EM07_InterlockVtg>"

== system edrive/Motor Control Board/GTM ==
  stGateDrv : Inport
  tSwitch : Inport  Port=2
  flgReqSafeSt : Inport  Port=3
  ASC : Constant  Value=[0 1 0 1 0 1]  SampleTime=-1
  Bus Selector1 : BusSelector  OutputSignals=SSM_flgReqSafeSt
  Constant : Constant  OutDataTypeStr=uint16
  DTC8 : DataTypeConversion  OutDataTypeStr=double
  FWL : Constant  Value=[0 0 0 0 0 0]  SampleTime=-1
  Multiport Switch : MultiPortSwitch  DataPortOrder=Specify indices  DataPortIndices={EGM.Freewheel,EGM.Shortcircuit, EGM.ShortcircuitTop, EGM.PWMRun, EGM.PWMDischarge}  DataPortForDefault=Additional data port
      settings: AttributesFormatString=|
      | ------------------------------
      | pwm discharge disabled temperary
  Multiport Switch1 : MultiPortSwitch  DataPortOrder=Specify indices  DataPortIndices={EGM.Freewheel,EGM.Shortcircuit, EGM.ShortcircuitTop, EGM.PWMRun, EGM.PWMDischarge}  DataPortForDefault=Additional data port
      settings: AttributesFormatString=|
      | ------------------------------
      | ASC preferred. FWL and oASC supported
  RateTransition1 : RateTransition
  RateTransition2 : RateTransition
  RateTransition4 : RateTransition  X0=EGM.Shortcircuit
  SVPWMtoDuty : Subsystem  AncestorBlock=|  DialogController=POWERSYS.PowerSysDialog  TreatAsAtomicUnit=on  mask(Discrete SV PWM Generator){InputType=alpha-beta components, SwitchingPattern=Pattern #1, Fc=1/Tsw, ParUref=[0.8 -30 50], Ts=-1}
      | powerlib_extras/Discrete 
      | Control Blocks/Discrete SV PWM
      | Generator
      mask prompts: InputType "Data type of input reference vector (U*):"; SwitchingPattern "Switching pattern:"; Fc "Chopping frequency (Hz):"; ParUref "Output voltage: [ Mag(0<m<1) Phase(deg.)  Freq(Hz) ]"; Ts "Sample time:"
      mask help:
      | This block generates pulses for a three-phase basic two-level voltage-sourced converter (VSC) consisting of three half-bridge switching devices (FETs, GTOs or IGBTs).
      | The block utilizes the space vector pulse width modulation (SV PWM) technique to generate firing pulses to the 6 switching devices of the converter. Two switching patterns can be selected.
      | The modulation index m (magnitude of the reference vector U) must be a value between 0 and 1.
      | The line-to-line rms voltage generated by a VSC controlled by this block will be: Vout= m * Vdc / sqrt(2).
      mask init:
      | powericon('DSVPWMGeneratorCback',gcb);
      | m=ParUref(1);
      | Pha=ParUref(2);
      | Freq=ParUref(3);
      | power_initmask();
      mask Help: This block is part of a subset of blocks in the Extras library that does not have documentation associated with it, other than the block mask description.
      mask TypeOptions InputType: Magnitude-Angle (rad) | alpha-beta components | Internally generated
      mask Callback InputType: %powericon('DSVPWMGeneratorCback',gcb);
      mask TypeOptions SwitchingPattern: Pattern #1 | Pattern #2
      mask Display: disp('')
  Sum : Sum  Inputs=|++
  Switch1 : Switch  Criteria=u2 > Threshold
  oASC : Constant  Value=[1 0 1 0 1 0]  SampleTime=-1
  time : Gain  Gain=1e-8
  PWM_Out : Outport
  wires:
  time/1 -> RateTransition1/1
  DTC8/1 -> time/1
  SVPWMtoDuty/1(Pulses) -> Multiport Switch/5
  RateTransition1/1 -> SVPWMtoDuty/1(tSwitch)
  RateTransition2/1 -> Switch1/2
  RateTransition4/1 -> Multiport Switch/1, Multiport Switch1/1
  Sum/1 -> DTC8/1
  ASC/1 -> Switch1/1, Multiport Switch1/3, Multiport Switch1/5, Multiport Switch/3
  oASC/1 -> Multiport Switch1/4, Multiport Switch/4
  FWL/1 -> Multiport Switch/7, Multiport Switch/6, Multiport Switch/2, Multiport Switch1/7, Multiport Switch1/6, Multiport Switch1/2
  Multiport Switch/1 -> Switch1/3
  Switch1/1 -> PWM_Out/1
  stGateDrv/1 -> RateTransition4/1
  tSwitch/1 -> Sum/1
  Constant/1 -> Sum/2
  Bus Selector1/1 -> RateTransition2/1  "<SSM_flgReqSafeSt>"
  flgReqSafeSt/1 -> Bus Selector1/1

== system edrive/Motor Control Board/Hardware platform ==
  10ms0to2 : Inport
  1ms0to2 : Inport  Port=2
  DO : Inport  Port=3
  10ms2to0 : Inport  Port=4
  Lv1_NESO : Inport  Port=5
  Lv2_ASCEN : Inport  Port=6
  Lv3_NERROR : Inport  Port=7
  Bus Creator : BusCreator  Inputs=15
  Bus Creator1 : BusCreator  Inputs=2
  Bus Selector : BusSelector  OutputSignals=MR,ENSMPS,ENL,ENH
  Bus Selector1 : BusSelector  OutputSignals=SSM_bRelsHiDfw,SSM_bRelsLoDfw,SSM_ModHiIgbtDrv,SSM_ModLoIgbtDrv
  Bus Selector2 : BusSelector  OutputSignals=NESO
  Logical Operator : Logic  AllPortsSameDT=off  OutDataTypeStr=boolean
  Logical Operator1 : Logic  Operator=NOT  AllPortsSameDT=off  OutDataTypeStr=boolean
  Motor Control Board : MATLAB Function
  RateTransition1 : RateTransition  OutPortSampleTime=ctrlConst.TsSim
  RateTransition2 : RateTransition  OutPortSampleTime=ctrlConst.TsSim
  RateTransition4 : RateTransition  OutPortSampleTime=ctrlConst.TsSim
  toInput : Outport
  toOutput : Outport  Port=2
  wires:
  DO/1 -> RateTransition1/1, RateTransition4/1
  Bus Creator/1 -> toInput/1
  Motor Control Board/1(KL30) -> Bus Creator/1  "KL30"
  Motor Control Board/2(KL30_1) -> Bus Creator/2  "KL30_1"
  Motor Control Board/3(VDD15) -> Bus Creator/3  "Vdd15"
  Motor Control Board/4(VDD15Fb) -> Bus Creator/4  "Vdd15FB"
  RateTransition4/1 -> Bus Selector/1
  Bus Selector1/2 -> Motor Control Board/6(RelsLoDfw)  "<SSM_bRelsLoDfw>"
  Bus Selector1/1 -> Motor Control Board/5(RelsHiDfw)  "<SSM_bRelsHiDfw>"
  Motor Control Board/5(RDY_H) -> Bus Creator/5  "RDY_H"
  Motor Control Board/6(RDY_L) -> Bus Creator/6  "RDY_L"
  1ms0to2/1 -> RateTransition2/1
  RateTransition2/1 -> Bus Selector1/1
  Bus Selector1/3 -> Motor Control Board/7(modHiIgbtDrv)  "<SSM_ModHiIgbtDrv>"
  Bus Selector1/4 -> Motor Control Board/8(modLoIgbtDrv)  "<SSM_ModLoIgbtDrv>"
  Motor Control Board/11(modIgbtDrvL2) -> Bus Creator/11  "modIgbtDrvL2"
  Motor Control Board/12(modIgbtDrvL3) -> Bus Creator/12  "modIgbtDrvL3"
  Motor Control Board/10(modIgbtDrvL1) -> Bus Creator/10  "modIgbtDrvL1"
  Motor Control Board/14(modIgbtDrvH2) -> Bus Creator/14  "modIgbtDrvH2"
  Motor Control Board/13(modIgbtDrvH1) -> Bus Creator/13  "modIgbtDrvH1"
  Motor Control Board/15(modIgbtDrvH3) -> Bus Creator/15  "modIgbtDrvH3"
  Motor Control Board/7(LvMoCSOP) -> Bus Creator/7  "LvMoCSOP"
  Motor Control Board/8(HvMoCSOP) -> Bus Creator/8  "HvMoCSOP"
  Lv3_NERROR/1 -> Logical Operator/2
  Logical Operator/1 -> Logical Operator1/1
  Bus Creator1/1 -> toOutput/1
  Logical Operator1/1 -> Bus Creator1/1  "Hw_Emgy_ASC"
  Lv2_ASCEN/1 -> Bus Creator1/2  "Lv2_ASCEN"
  Motor Control Board/9(stIgbtDrvCnfgOk) -> Bus Creator/9
  Bus Selector/1 -> Motor Control Board/1(MR_ON)  "<MR>"
  Bus Selector/2 -> Motor Control Board/2(bCtlSmps)  "<ENSMPS>"
  Bus Selector/3 -> Motor Control Board/3(bLoEnFen)  "<ENL>"
  Bus Selector/4 -> Motor Control Board/4(bHiEnFen)  "<ENH>"
  RateTransition1/1 -> Bus Selector2/1
  Lv1_NESO/1 -> Logical Operator/1

== system edrive/Motor Control Board/IGBT Driver ==
  PWM_In : Inport
  Emgy_ASC : Inport  Port=2
  Bus Selector1 : BusSelector  OutputSignals=Hw_Emgy_ASC,Lv2_ASCEN
  LoASC : Constant  Value=[0 1 0 1 0 1]  SampleTime=-1
  Logical Operator : Logic  Operator=OR  AllPortsSameDT=off  OutDataTypeStr=boolean
  RateTransition2 : RateTransition  X0=true
  Switch1 : Switch  Criteria=u2 > Threshold  Threshold=0.5
  PWM_Out : Outport
  wires:
  RateTransition2/1 -> Switch1/2
  LoASC/1 -> Switch1/1
  PWM_In/1 -> Switch1/3
  Switch1/1 -> PWM_Out/1
  Emgy_ASC/1 -> Bus Selector1/1
  Bus Selector1/1 -> Logical Operator/1  "<Hw_Emgy_ASC>"
  Bus Selector1/2 -> Logical Operator/2  "<Lv2_ASCEN>"
  Logical Operator/1 -> RateTransition2/1
